simulink model "511743_exp4_pi.sim"  (R2015a)
settings: Solver=ode15s  StartTime=0.0  StopTime=0.002  MaxStep=0.00002  RelTol=1e-3
libraries: fl_lib x9, nesl_utility x3
Description:
  | Differentiator
  | 
  | This model shows a differentiator, such as might be used as part
  | of a PID controller. It also illustrates how numerical simulation issues
  | can arise in some idealized circuits. The model runs with the
  | capacitor series parasitic resistance set to its default value of 1e-6
  | Ohms. Setting it to zero results in a warning and a very slow
  | simulation. See the User's Guide for further information.
  | 
  | 
  | Copyright 2008-2015 The MathWorks, Inc.
settings Model: ExtModeAutoUpdateStatusClock=off  Creator=MathWorks  LastModifiedBy=vikas
settings DataIOCC: SignalLoggingSaveFormat=ModelDataLogs
settings OptimizationCC: ExpressionDepthLimit=2147483647  InitFltsAndDblsToZero=on
settings DebuggingCC: SaveWithParameterizedLinksMsg=none  UnderspecifiedInitializationDetection=Classic  MergeDetectMultiDrivingBlocksExec=none  SignalResolutionControl=TryResolveAllWithWarning  SolverPrmCheckMsg=warning  FcnCallInpInsideContextMsg=UseLocalSettings  StateNameClashWarn=warning
settings GRTTargetCC: TargetFcnLib=ansi_tfl_tmw.mat  CombineOutputUpdateFcns=off  GRTInterface=on

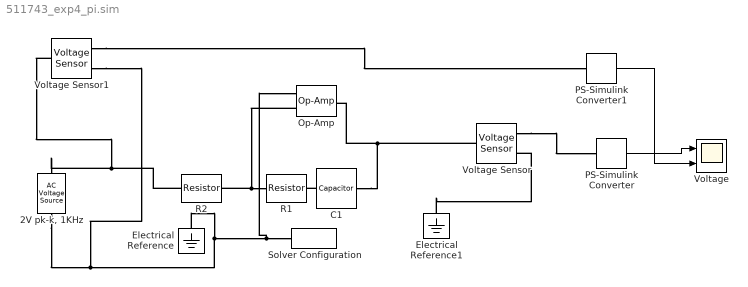
== system 511743_exp4_pi.sim ==
  "2V pk-k, 1KHz" : fl_lib/Electrical/Electrical Sources/AC Voltage Source  amp=1 V  shift=0 deg  frequency=1000 Hz  omega=0 rad/s
  C1 : fl_lib/Electrical/Electrical Elements/Capacitor  c=1/(10e3*2*pi*1000) F  r=1e-6 Ohm  g=0 1/Ohm  i_specify=off  i_priority=High  i=0 A  v_specify=off  v_priority=High  v=0 V  vc_specify=on  vc_priority=High  vc=0 V
  Electrical Reference : fl_lib/Electrical/Electrical Elements/Electrical Reference
  Electrical Reference1 : fl_lib/Electrical/Electrical Elements/Electrical Reference
  Op-Amp : fl_lib/Electrical/Electrical Elements/Op-Amp  outI_specify=off  outI_priority=High  outI=0 A
  PS-Simulink Converter : nesl_utility/PS-Simulink Converter  PhysicalDomain=network_engine_domain  SubClassName=ps_output  LeftPortType=input  RightPortType=output  PseudoPeriodic=off  Frequencies=[]  Unit=1  AffineConversion=off
  PS-Simulink Converter1 : nesl_utility/PS-Simulink Converter  PhysicalDomain=network_engine_domain  SubClassName=ps_output  LeftPortType=input  RightPortType=output  PseudoPeriodic=off  Frequencies=[]  Unit=1  AffineConversion=off
  R1 : fl_lib/Electrical/Electrical Elements/Resistor  R=500 Ohm  i_specify=off  i_priority=High  i=0 A  v_specify=off  v_priority=High  v=0 V
  R2 : fl_lib/Electrical/Electrical Elements/Resistor  R=1000 Ohm  i_specify=off  i_priority=High  i=0 A  v_specify=off  v_priority=High  v=0 V
  Solver Configuration : nesl_utility/Solver Configuration  PhysicalDomain=network_engine_domain  SubClassName=solver  LeftPortType=input  RightPortType=generic  Accelerate=off  Tones=[]  Harmonics=[]  SimulateNoise=off  Profile=off  UseLocalSampling=off  EnableSwitchedLinearOptims=on  FrequencyDomain=off  UseCCode=off  RelTol=0.001  AbsTol=1e-06  MinStep=1e-09  ToWorkspace=off  RevertToSquareIcSolve=off  NumHomotopyIterations=100  DoDC=off  ResidualTolerance=1e-9  UseLocalSolver=off  LocalSolverChoice=NE_BACKWARD_EULER_ADVANCER  LocalSolverSampleTime=.001  DoFixedCost=off  MaxNonlinIter=3  MaxModeIter=2  LinearAlgebra=Sparse  DelaysMemoryBudget=1024  AutomaticFiltering=on  FilteringTimeConstant=0.001
  Voltage : Scope  NumInputPorts=2
      settings: YMin=-2~-5  YMax=2~5
  Voltage Sensor : fl_lib/Electrical/Electrical Sensors/Voltage Sensor
  Voltage Sensor1 : fl_lib/Electrical/Electrical Sensors/Voltage Sensor
  wires:
  PS-Simulink Converter/1 -> Voltage/1
  PS-Simulink Converter1/1 -> Voltage/2
  connections:
  Voltage Sensor1/RConn2 -- "2V pk-k, 1KHz"/RConn1 -- Electrical Reference/LConn1 -- Op-Amp/LConn1 -- Solver Configuration/RConn1
  "2V pk-k, 1KHz"/LConn1 -- R2/LConn1 -- Voltage Sensor1/LConn1
  Op-Amp/LConn2 -- R2/RConn1 -- R1/LConn1
  Voltage Sensor/LConn1 -- C1/RConn1 -- Op-Amp/RConn1
  Electrical Reference1/LConn1 -- Voltage Sensor/RConn2
  Voltage Sensor/RConn1 -- PS-Simulink Converter/LConn1
  C1/LConn1 -- R1/RConn1
  Voltage Sensor1/RConn1 -- PS-Simulink Converter1/LConn1
